simulink model "m2asm_2_rust"  (R2020b)
settings: Solver=FixedStepDiscrete  StartTime=0.0  StopTime=5  FixedStep=deltaT  RelTol=1e-3
InitFcn:
  | %
  | % Initialization callback function
  | %
  | 
  | try
  |    fprintf('\n New GMT IMS version!\n');
  | 
  |    % Get Simulink model directory
  |    [filepath,name,ext] = fileparts(which(bdroot));
  | 
  |    if ~strcmp(filepath,pwd)
  |       fprintf('\n Changing current directory to \n %s \n',filepath);
  |       cd(filepath);
  |    end
  | 
  |    %
  |    if(~exist('IMLoads','var'))
  |        warning('Simulation model assumes wind load is loaded...');
  |    end
  | catch
  |    warning('Running the InitFcn from puSimulate script');
  | end
values from neighbouring files (symbols this model uses):
  Cpi_d = c2d(st.asm.fpi,Ts,c2d_opts)    [load_m2asm_data.m]
  flag_d = c2d(flag,Ts,c2d_opts)    [load_m2asm_data.m]
  Hpd_d = c2d(st.asm.fpd,Ts,c2d_opts)    [load_m2asm_data.m]
  st = getcontrol_asm()    [load_m2asm_data.m]
settings Model: SimulationMode=accelerator  Creator=RRomano  LastModifiedBy=rromano
settings DataIOCC: SaveOutput=off  SignalLogging=off  DSMLogging=off  SaveTime=off  ReturnWorkspaceOutputs=off
settings OptimizationCC: StrengthReduction=on  PassReuseOutputArgsAs=Individual arguments  EfficientMapNaN2IntZero=off  SimCompilerOptimization=on  AccelVerboseBuild=on  OptimizeBlockOrder=speed  OptimizationPriority=Speed  OptimizationCustomize=off  MultiThreadedLoops=on  EfficientTunableParamExpr=on
settings DebuggingCC: InheritedTsInSrcMsg=none  MultiTaskRateTransMsg=warning  ParameterTunabilityLossMsg=error  SFUnexpectedBacktrackingDiag=warning  SFNoUnconditionalDefaultTransitionDiag=warning  SFExecutionAtInitializationDiag=none  ArithmeticOperatorsInVariantConditions=warning
settings HardwareCC: ProdBitPerLong=64  ProdHWDeviceType=Intel->x86-64 (Linux 64)  TargetBitPerLong=64  TargetBitPerPointer=64  TargetBitPerSizeT=64  TargetBitPerPtrDiffT=64  TargetLongLongMode=on  TargetIntDivRoundTo=Zero  TargetEndianess=LittleEndian  TargetWordSize=64  TargetHWDeviceType=MATLAB Host  ProdEqTarget=off
settings SFSimCC: SimUseLocalCustomCode=off  MATLABDynamicMemAlloc=off  CustomCodeUndefinedFunction=UseInterfaceOnly
settings RTWCC: Description=Embedded Coder  SystemTargetFile=ert.tlc  GenCodeOnly=on  TemplateMakefile=ert_default_tmf  GenerateReport=on  BuildConfiguration=Faster Runs  IncludeHyperlinkInReport=on  GenerateTraceInfo=on  GenerateTraceReport=on  GenerateTraceReportSl=on  GenerateTraceReportSf=on  GenerateTraceReportEml=on
settings CodeAppCC: ForceParamTrailComments=on  IgnoreCustomStorageClasses=off  MaxIdLength=128  OperatorAnnotations=on  SimulinkDataObjDesc=on  SFDataObjDesc=on  InsertBlockDesc=on  MATLABSourceComments=on
settings ERTTargetCC: GenerateSampleERTMain=on  SuppressErrorStatus=on  CodeInterfacePackaging=Reusable function  RootIOFormat=Structure reference  ERTCustomFileTemplate=example_file_process.tlc
settings ConfigComp: CovMetricSettings=dw  CovSaveCumulativeToWorkspaceVar=on  CovSaveSingleToWorkspaceVar=on  CovExternalEMLEnable=off

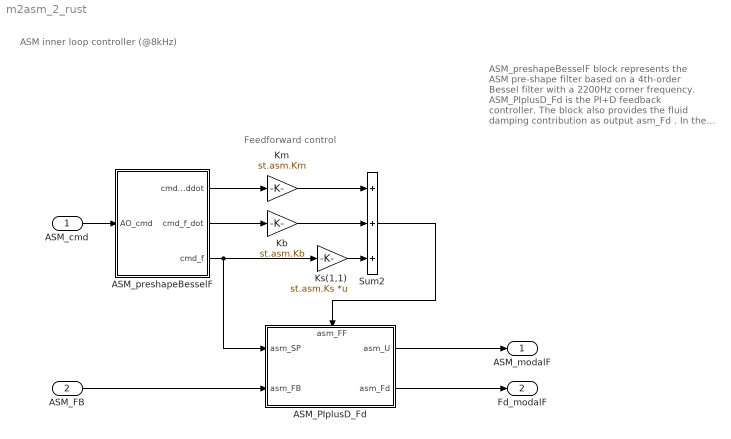
== system m2asm_2_rust ==
  note: Feedforward control
  note: ASM_preshapeBesselF block represents the ASM pre-shape filter based on a 4th-order Bessel filter with a 2200Hz corner frequency.
      | ASM_PIplusD_Fd is the PI+D feedback controller. The block also provides the fluid damping contribution as output asm_Fd .
      | In the modal control approach, Ks is the inverse of the modal stiffness matrix, a square matrix of dimension n_m. Therefore, in that case, Ks(1,1) is just a placeholder.
  note: ASM inner loop controller (@8kHz)
  ASM_cmd : Inport  Interpolate=off
  ASM_FB : Inport  Port=2
  ASM_PIplusD_Fd : Subsystem
      settings: PortSchema="{\"entries\":[{\"content\":{\"sides\":[{\"content\":{\"connectorIds\":[\"In1\",\"In2\"]},\"type\":\"ConnectorPlacement.EquallySpacedRectSide\",\"uuid\":\"706a4ecf-f719-44ad-a306-9c11e57cb316\"},{\"content\":{\"connectorIds\":[\"Out1\",\"Out2\"],\"side\":\"RIGHT\"},\"type\":\"ConnectorPlacement.EquallySpacedRectSide\",\"uuid\":\"04f8501d-a7a5-4c7b-93f1-e2b34d7c8dac\"},{\"content\":{\"connectorIds\":[\"In3\"],\"side\":\"TOP\"},\"type\":\"ConnectorPlacement.EquallySpacedRectSide\",\"uuid\":\"7dc3ff34-2b4e-4efd-8743-462d0862980d\"},{\"content\":{\"connectorIds\":[],\"side\":\"HIDDEN\"},\"type\":\"ConnectorPlacement.EquallySpacedRectSide\",\"uuid\":\"673e63a6-b266-47a9-b9c4-9219546d9f5b\"}]},\"type\":\"ConnectorPlacement.EquallySpacedConnector\",\"uuid\":\"903795e5-c455-47ea-8916-0bf0c79c1da5\"}],\"packageUris\":[\"http://schema.mathworks.com/mf0/Connector/R2020b\"],\"version\":\"1.0\"}"
  ASM_preshapeBesselF : Subsystem
  Kb : Gain  Gain=st.asm.Kb
  Km : Gain  Gain=st.asm.Km
  Ks(1,1) : Gain  Gain=st.asm.Ks  Multiplication=Matrix(K*u)
  Sum2 : Sum  Inputs=+++
  ASM_modalF : Outport  VectorParamsAs1DForOutWhenUnconnected=off
  Fd_modalF : Outport  Port=2  VectorParamsAs1DForOutWhenUnconnected=off
  wires:
  ASM_PIplusD_Fd/1(asm_U) -> ASM_modalF/1
  Sum2/1 -> ASM_PIplusD_Fd/3(asm_FF)
  Km/1 -> Sum2/1
  Kb/1 -> Sum2/2
  Ks(1,1)/1 -> Sum2/3
  ASM_cmd/1 -> ASM_preshapeBesselF/1(AO_cmd)
  ASM_preshapeBesselF/3(cmd_f) -> ASM_PIplusD_Fd/1(asm_SP), Ks(1,1)/1
  ASM_preshapeBesselF/2(cmd_f_dot) -> Kb/1
  ASM_FB/1 -> ASM_PIplusD_Fd/2(asm_FB)
  ASM_PIplusD_Fd/2(asm_Fd) -> Fd_modalF/1
  ASM_preshapeBesselF/1(cmd_f_ddot) -> Km/1

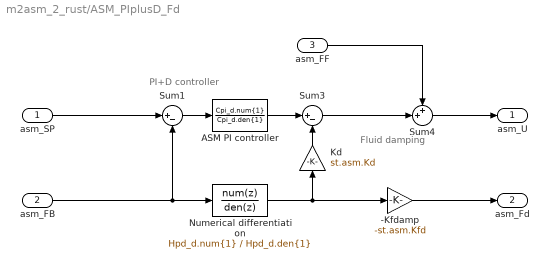
== system m2asm_2_rust/ASM_PIplusD_Fd ==
  note: PI+D controller
  note: Fluid damping
  asm_SP : Inport
  asm_FB : Inport  Port=2
  asm_FF : Inport  Port=3
  -Kfdamp : Gain  Gain=-st.asm.Kfd
  ASM PI controller : DiscreteTransferFcn  Numerator=Cpi_d.num{1}  Denominator=Cpi_d.den{1}  SampleTime=Cpi_d.Ts
  Kd : Gain  Gain=st.asm.Kd
  Numerical differentiation : DiscreteTransferFcn  Numerator=Hpd_d.num{1}  Denominator=Hpd_d.den{1}  SampleTime=Hpd_d.Ts
  Sum1 : Sum  Inputs=|+-
  Sum3 : Sum  Inputs=|+-
  Sum4 : Sum  Inputs=++|
  asm_U : Outport
  asm_Fd : Outport  Port=2
  wires:
  Kd/1 -> Sum3/2
  ASM PI controller/1 -> Sum3/1
  asm_SP/1 -> Sum1/1
  Numerical differentiation/1 -> -Kfdamp/1, Kd/1
  asm_FB/1 -> Numerical differentiation/1, Sum1/2
  Sum1/1 -> ASM PI controller/1
  -Kfdamp/1 -> asm_Fd/1
  Sum3/1 -> Sum4/2
  asm_FF/1 -> Sum4/1
  Sum4/1 -> asm_U/1

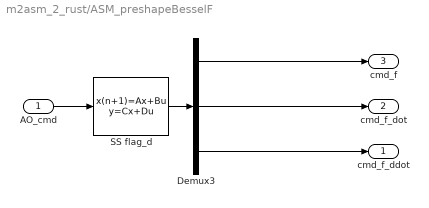
== system m2asm_2_rust/ASM_preshapeBesselF ==
  AO_cmd : Inport
  Demux3 : Demux  Outputs=3
  SS flag_d : DiscreteStateSpace  A=flag_d.A  B=flag_d.B  C=flag_d.C  D=flag_d.D  SampleTime=flag_d.Ts
  cmd_f_ddot : Outport
  cmd_f_dot : Outport  Port=2
  cmd_f : Outport  Port=3
  wires:
  Demux3/1 -> cmd_f/1
  Demux3/3 -> cmd_f_ddot/1
  Demux3/2 -> cmd_f_dot/1
  AO_cmd/1 -> SS flag_d/1
  SS flag_d/1 -> Demux3/1
